simulink model "ball_and_beam_simulink"  (R2014b)
settings: Solver=ode45  StartTime=0.0  StopTime=10  RelTol=1e-3
values from neighbouring files (symbols this model uses):
  Bm = 0.01    [ball.m]    (also in ball_and_beam.m; tham_so.m)
  d = 0.02    [ball.m]    (also in ball_and_beam.m = 0.04; draft.m; parameter.m = 0.04)
  g = 9.8    [ball.m]    (also in ball_and_beam.m; tham_so.m)
  h = 0.08    [ball.m]    (also in ball_and_beam.m; draft.m)
  h1 = 0.0    (= 0)    [ball.m]    (also in draft.m)
  JB = (2/5)*mB*rB^2    (= 1.0469e-06)    [ball.m]    (also in ball_and_beam.m; parameter.m = (2/5)*mB*R^2; tham_so.m)
  Jm = 0.000052    (= 5.2e-05)    [ball.m]    (also in ball_and_beam.m; tham_so.m)
  k = 0.08    [ball.m]    (also in ball_and_beam.m = 0.12; draft.m)
  Ke = 0.235    [ball.m]    (also in ball_and_beam.m; tham_so.m)
  Kt = 0.235    [ball.m]    (also in ball_and_beam.m; tham_so.m)
  l = 0.4    [ball.m]    (also in ball_and_beam.m; draft.m)
  La = 0.23    [ball.m]    (also in ball_and_beam.m; tham_so.m)
  mB = 0.029    [ball.m]    (also in ball_and_beam.m; parameter.m; tham_so.m)
  Ra = 2    [ball.m]    (also in ball_and_beam.m; tham_so.m)
  rB = 0.0095    [ball.m]    (also in ball_and_beam.m; tham_so.m)
  xd = 0.4 - d    (= 0.38)    [ball.m]    (also in ball_and_beam.m = 0.36; draft.m)
settings Model: Creator=nghia  LastModifiedBy=Admin

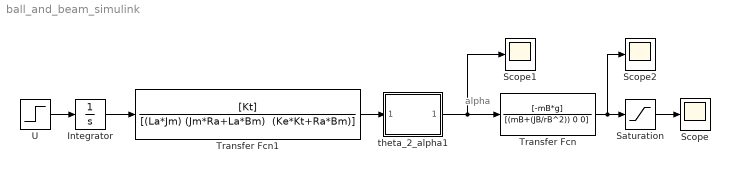
== system ball_and_beam_simulink ==
  note: alpha
  Integrator : Integrator
  Saturation : Saturate  UpperLimit=l  LowerLimit=0
  Scope : Scope
      settings: TimeRange=10  YMin=-1  YMax=1
  Scope1 : Scope
      settings: TimeRange=10  YMin=-140  YMax=0
  Scope2 : Scope
      settings: TimeRange=10  YMin=-140  YMax=0  SaveName=ScopeData2
  Transfer Fcn : TransferFcn  Numerator=[-mB*g]  Denominator=[(mB+(JB/rB^2)) 0 0]
  Transfer Fcn1 : TransferFcn  Numerator=[Kt]  Denominator="[(La*Jm) (Jm*Ra+La*Bm)  (Ke*Kt+Ra*Bm)]"
  U : Step  Time=0  SampleTime=0
  theta_2_alpha1 : Subsystem
  wires:
  Transfer Fcn1/1 -> theta_2_alpha1/1(theta)
  theta_2_alpha1/1(alpha) -> Transfer Fcn/1, Scope1/1
  Integrator/1 -> Transfer Fcn1/1
  U/1 -> Integrator/1
  Transfer Fcn/1 -> Scope2/1, Saturation/1
  Saturation/1 -> Scope/1

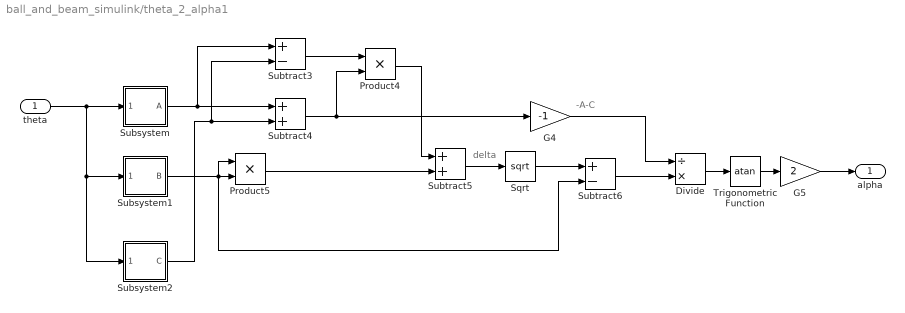
== system ball_and_beam_simulink/theta_2_alpha1 ==
  note: -A-C
  note: delta
  theta : Inport
  Divide : Product  Inputs=/*
  G4 : Gain  Gain=-1
  G5 : Gain  Gain=2
  Product4 : Product
  Product5 : Product
  Sqrt : Sqrt  SaturateOnIntegerOverflow=on
  Subsystem : Subsystem
  Subsystem1 : Subsystem
  Subsystem2 : Subsystem
  Subtract3 : Sum  Inputs=+-
  Subtract4 : Sum
  Subtract5 : Sum
  Subtract6 : Sum  Inputs=+-
  Trigonometric Function : Trigonometry  Operator=atan
  alpha : Outport
  wires:
  Divide/1 -> Trigonometric Function/1
  G5/1 -> alpha/1
  Subtract5/1 -> Sqrt/1
  Product5/1 -> Subtract5/2
  Subtract3/1 -> Product4/1
  Trigonometric Function/1 -> G5/1
  Product4/1 -> Subtract5/1
  Sqrt/1 -> Subtract6/1
  Subtract4/1 -> G4/1, Product4/2
  theta/1 -> Subsystem2/1(theta), Subsystem1/1(theta), Subsystem/1(theta)
  Subsystem1/1(B) -> Subtract6/2, Product5/1, Product5/2
  Subsystem/1(A) -> Subtract3/1, Subtract4/1
  Subsystem2/1(C) -> Subtract3/2, Subtract4/2
  G4/1 -> Divide/1
  Subtract6/1 -> Divide/2

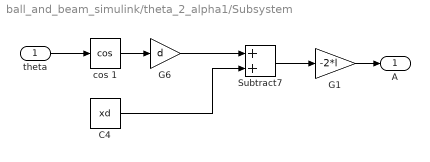
== system ball_and_beam_simulink/theta_2_alpha1/Subsystem ==
  theta : Inport
  C4 : Constant  Value=xd
  G1 : Gain  Gain=-2*l
  G6 : Gain  Gain=d
  Subtract7 : Sum
  cos 1 : Trigonometry  Operator=cos
  A : Outport
  wires:
  Subtract7/1 -> G1/1
  G6/1 -> Subtract7/1
  C4/1 -> Subtract7/2
  cos 1/1 -> G6/1
  theta/1 -> cos 1/1
  G1/1 -> A/1

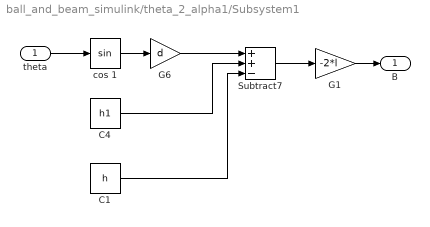
== system ball_and_beam_simulink/theta_2_alpha1/Subsystem1 ==
  theta : Inport
  C1 : Constant  Value=h
  C4 : Constant  Value=h1
  G1 : Gain  Gain=-2*l
  G6 : Gain  Gain=d
  Subtract7 : Sum  Inputs=++-
  cos 1 : Trigonometry
  B : Outport
  wires:
  Subtract7/1 -> G1/1
  G6/1 -> Subtract7/1
  C4/1 -> Subtract7/2
  cos 1/1 -> G6/1
  theta/1 -> cos 1/1
  G1/1 -> B/1
  C1/1 -> Subtract7/3

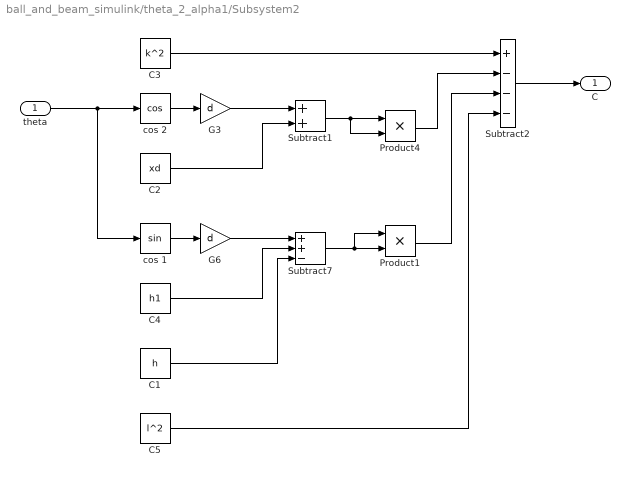
== system ball_and_beam_simulink/theta_2_alpha1/Subsystem2 ==
  theta : Inport
  C1 : Constant  Value=h
  C2 : Constant  Value=xd
  C3 : Constant  Value=k^2
  C4 : Constant  Value=h1
  C5 : Constant  Value=l^2
  G3 : Gain  Gain=d
  G6 : Gain  Gain=d
  Product1 : Product
  Product4 : Product
  Subtract1 : Sum
  Subtract2 : Sum  Inputs=+---
  Subtract7 : Sum  Inputs=++-
  cos 1 : Trigonometry
  cos 2 : Trigonometry  Operator=cos
  C : Outport
  wires:
  G6/1 -> Subtract7/1
  C4/1 -> Subtract7/2
  cos 1/1 -> G6/1
  C1/1 -> Subtract7/3
  G3/1 -> Subtract1/1
  C2/1 -> Subtract1/2
  cos 2/1 -> G3/1
  Subtract2/1 -> C/1
  C3/1 -> Subtract2/1
  Subtract1/1 -> Product4/2, Product4/1
  Product4/1 -> Subtract2/2
  Subtract7/1 -> Product1/2, Product1/1
  Product1/1 -> Subtract2/3
  C5/1 -> Subtract2/4
  theta/1 -> cos 1/1, cos 2/1
